simulink subsystem "Global_to_Local_WayPoints"  (R2022b)
settings: Solver=VariableStepAuto  StartTime=0.0  StopTime=10.0  RelTol=1e-3
settings Model: Creator=User  LastModifiedBy=User

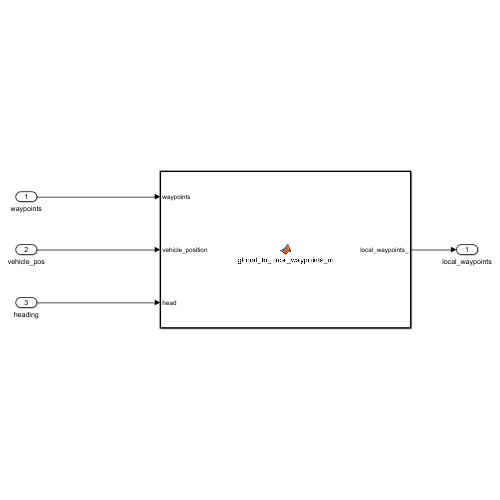
[thumbnail: Simulink's stored preview of the top-level diagram]
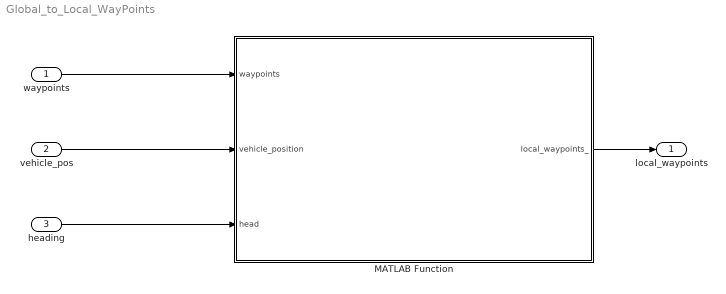
== system Global_to_Local_WayPoints ==
  waypoints : Inport
  vehicle_pos : Inport  Port=2
  heading : Inport  Port=3
  MATLAB Function : MATLAB Function  TreatAsAtomicUnit=on
  local_waypoints : Outport
  wires:
  waypoints/1 -> MATLAB Function/1(waypoints)
  vehicle_pos/1 -> MATLAB Function/2(vehicle_position)
  heading/1 -> MATLAB Function/3(head)
  MATLAB Function/1(local_waypoints_) -> local_waypoints/1

== matlab function Global_to_Local_WayPoints/MATLAB Function ==
  data: waypoints input; local_waypoints_ output; vehicle_position input; head input
function local_waypoints_ = global_to_local_waypoints_m(waypoints, vehicle_position, head)
   local_waypoints_ = global_to_local_waypoints(waypoints, vehicle_position, head);
    
end
